simulink model "flatnessLinearNonLinear"  (R2023b)
settings: Solver=FixedStepAuto  StartTime=0.0  StopTime=7  RelTol=1e-3
model workspace (MAT data in the model file):
  kp = Simulink.Parameter
  kp.DataType = 'auto'
  kp.Complexity = 'real'
  kp.Dimensions = [0 0]
libraries: robotmobilelib x2, simulink x1
settings Model: Creator=RichiRettore  LastModifiedBy=RichiRettore

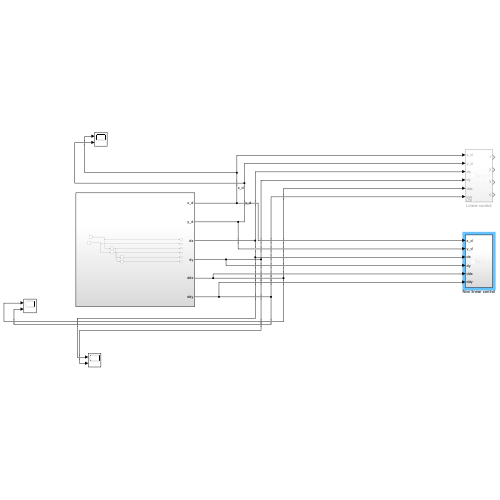
[thumbnail: Simulink's stored preview of the top-level diagram]
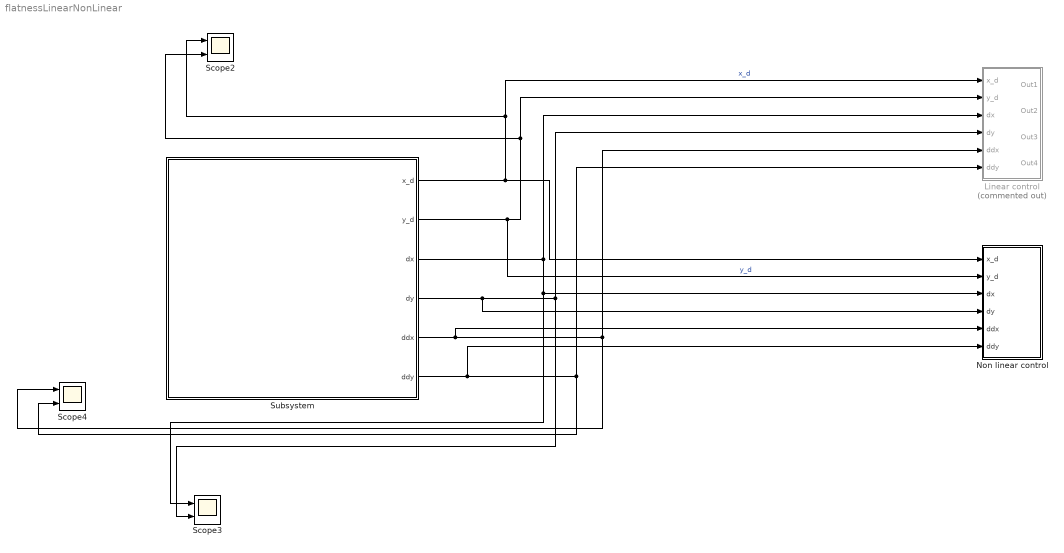
== system flatnessLinearNonLinear ==
  Linear control : Subsystem  Commented=on
  Non linear control : Subsystem
  Scope2 : Scope  NumInputPorts=2
  Scope3 : Scope  NumInputPorts=2
  Scope4 : Scope  NumInputPorts=2
  Subsystem : Subsystem
  wires:
  Subsystem/1(x_d) -> Non linear control/1(x_d), Linear control/1(x_d), Scope2/1  "x_d"
  Subsystem/2(y_d) -> Non linear control/2(y_d), Linear control/2(y_d), Scope2/2  "y_d"
  Subsystem/3(dx) -> Non linear control/3(dx), Scope3/1, Linear control/3(dx)
  Subsystem/4(dy) -> Non linear control/4(dy), Linear control/4(dy), Scope3/2
  Subsystem/5(ddx) -> Non linear control/5(ddx), Linear control/5(ddx), Scope4/1
  Subsystem/6(ddy) -> Non linear control/6(ddy), Linear control/6(ddy), Scope4/2

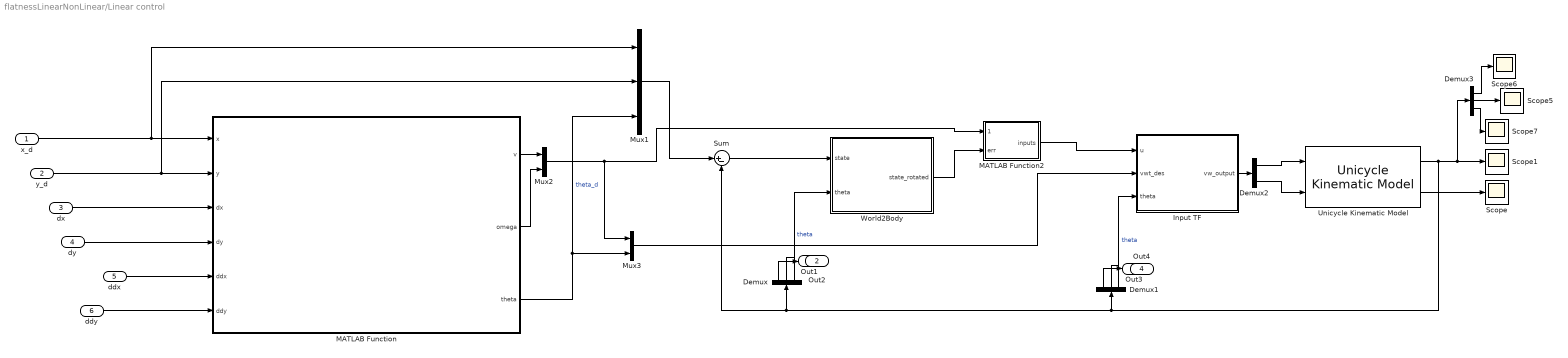
== system flatnessLinearNonLinear/Linear control ==
  x_d : Inport
  y_d : Inport  Port=2
  dx : Inport  Port=3
  dy : Inport  Port=4
  ddx : Inport  Port=5
  ddy : Inport  Port=6
  Demux : Demux  Outputs=3
  Demux1 : Demux  Outputs=3
  Demux2 : Demux  Outputs=2
  Demux3 : Demux  Outputs=3
  Input TF : MATLAB Function  TreatAsAtomicUnit=on
  MATLAB Function : MATLAB Function  TreatAsAtomicUnit=on
  MATLAB Function2 : MATLAB Function  TreatAsAtomicUnit=on
  Mux1 : Mux  Inputs=3
  Mux2 : Mux  Inputs=2
  Mux3 : Mux  Inputs=2
  Scope{,1,5..7} (5 alike) : Scope
  Sum : Sum  Inputs=|+-
  Unicycle Kinematic Model : robotmobilelib/Unicycle Kinematic Model  VehicleInputs=Vehicle Speed & Heading Angular Velocity  WheelRadius=0.1  WheelSpeedRange=[-Inf Inf]  InitialState=[1; 1; 1]  SimulateUsing=Interpreted execution
  World2Body : MATLAB Function  TreatAsAtomicUnit=on
  Out1 : Outport
  Out2 : Outport  Port=2
  Out3 : Outport  Port=3
  Out4 : Outport  Port=4
  wires:
  Demux1/3 -> Input TF/3(theta)  "theta"
  Unicycle Kinematic Model/1 -> Demux3/1, Scope1/1, Sum/2, Demux/1, Demux1/1
  MATLAB Function/2(omega) -> Mux2/2
  dx/1 -> MATLAB Function/3(dx)
  Demux/3 -> World2Body/2(theta)  "theta"
  x_d/1 -> Mux1/1, MATLAB Function/1(x)
  ddx/1 -> MATLAB Function/5(ddx)
  Sum/1 -> World2Body/1(state)
  World2Body/1(state_rotated) -> MATLAB Function2/2(err)
  Demux2/1 -> Unicycle Kinematic Model/1
  MATLAB Function2/1(inputs) -> Input TF/1(u)
  Demux2/2 -> Unicycle Kinematic Model/2
  Demux1/2 -> Out4/1
  Demux/2 -> Out2/1
  Input TF/1(vw_output) -> Demux2/1
  Mux1/1 -> Sum/1
  MATLAB Function/3(theta) -> Mux3/2, Mux1/3  "theta_d"
  y_d/1 -> Mux1/2, MATLAB Function/2(y)
  Demux3/1 -> Scope6/1
  Mux2/1 -> Mux3/1, MATLAB Function2/1(velocities)
  Mux3/1 -> Input TF/2(vwt_des)
  Demux3/3 -> Scope7/1
  Demux3/2 -> Scope5/1
  Unicycle Kinematic Model/2 -> Scope/1
  MATLAB Function/1(v) -> Mux2/1
  ddy/1 -> MATLAB Function/6(ddy)
  dy/1 -> MATLAB Function/4(dy)
  Demux1/1 -> Out3/1
  Demux/1 -> Out1/1

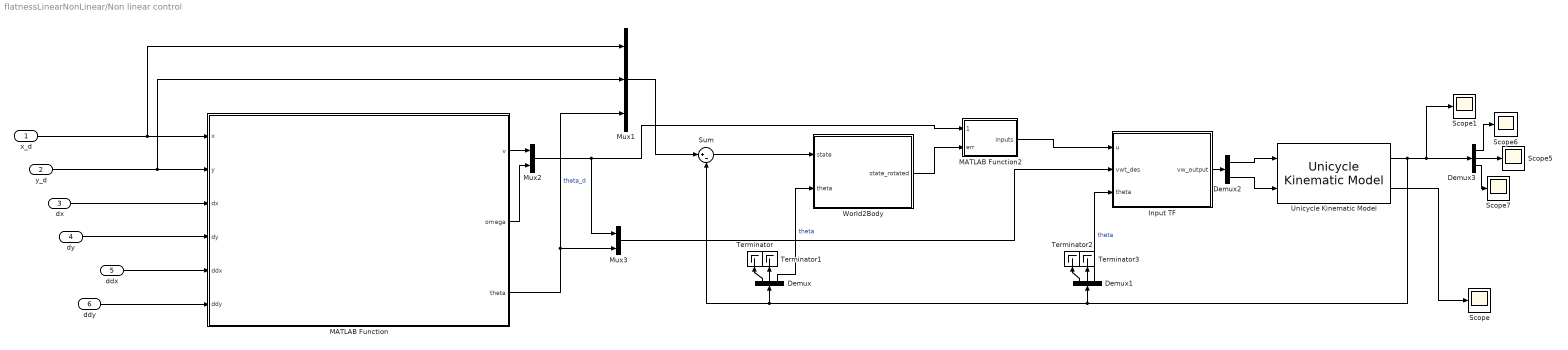
== system flatnessLinearNonLinear/Non linear control ==
  x_d : Inport
  y_d : Inport  Port=2
  dx : Inport  Port=3
  dy : Inport  Port=4
  ddx : Inport  Port=5
  ddy : Inport  Port=6
  Demux : Demux  Outputs=3
  Demux1 : Demux  Outputs=3
  Demux2 : Demux  Outputs=2
  Demux3 : Demux  Outputs=3
  Input TF : MATLAB Function  TreatAsAtomicUnit=on
  MATLAB Function : MATLAB Function  TreatAsAtomicUnit=on
  MATLAB Function2 : MATLAB Function  TreatAsAtomicUnit=on
  Mux1 : Mux  Inputs=3
  Mux2 : Mux  Inputs=2
  Mux3 : Mux  Inputs=2
  Scope{,1,5..7} (5 alike) : Scope
  Sum : Sum  Inputs=|+-
  Terminator{,1..3} (4 alike) : Terminator
  Unicycle Kinematic Model : robotmobilelib/Unicycle Kinematic Model  VehicleInputs=Vehicle Speed & Heading Angular Velocity  WheelRadius=0.1  WheelSpeedRange=[-Inf Inf]  InitialState=[1; 1; 1]  SimulateUsing=Interpreted execution
  World2Body : MATLAB Function  TreatAsAtomicUnit=on
  wires:
  Demux1/3 -> Input TF/3(theta)  "theta"
  Unicycle Kinematic Model/1 -> Demux3/1, Scope1/1, Sum/2, Demux/1, Demux1/1
  MATLAB Function/2(omega) -> Mux2/2
  dx/1 -> MATLAB Function/3(dx)
  Demux/3 -> World2Body/2(theta)  "theta"
  x_d/1 -> Mux1/1, MATLAB Function/1(x)
  ddx/1 -> MATLAB Function/5(ddx)
  Sum/1 -> World2Body/1(state)
  World2Body/1(state_rotated) -> MATLAB Function2/2(err)
  Demux2/1 -> Unicycle Kinematic Model/1
  MATLAB Function2/1(inputs) -> Input TF/1(u)
  Demux2/2 -> Unicycle Kinematic Model/2
  Input TF/1(vw_output) -> Demux2/1
  Mux1/1 -> Sum/1
  MATLAB Function/3(theta) -> Mux3/2, Mux1/3  "theta_d"
  y_d/1 -> Mux1/2, MATLAB Function/2(y)
  Demux3/1 -> Scope6/1
  Mux2/1 -> Mux3/1, MATLAB Function2/1(velocities)
  Mux3/1 -> Input TF/2(vwt_des)
  Demux3/3 -> Scope7/1
  Demux3/2 -> Scope5/1
  Unicycle Kinematic Model/2 -> Scope/1
  MATLAB Function/1(v) -> Mux2/1
  ddy/1 -> MATLAB Function/6(ddy)
  dy/1 -> MATLAB Function/4(dy)
  Demux/2 -> Terminator1/1
  Demux/1 -> Terminator/1
  Demux1/1 -> Terminator2/1
  Demux1/2 -> Terminator3/1

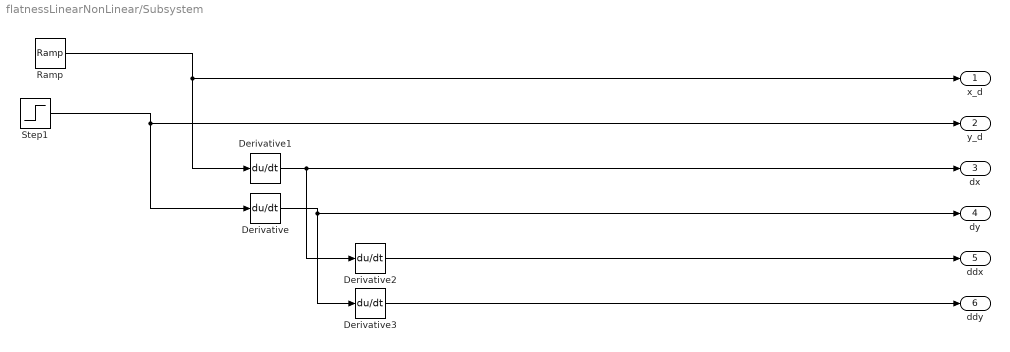
== system flatnessLinearNonLinear/Subsystem ==
  Derivative{,1..3} (4 alike) : Derivative
  Ramp : simulink/Sources/Ramp  slope=1  start=0  InitialOutput=0
  Step1 : Step  Time=0  After=5  SampleTime=0
  x_d : Outport
  y_d : Outport  Port=2
  dx : Outport  Port=3
  dy : Outport  Port=4
  ddx : Outport  Port=5
  ddy : Outport  Port=6
  wires:
  Derivative2/1 -> ddx/1
  Derivative1/1 -> Derivative2/1, dx/1
  Derivative/1 -> Derivative3/1, dy/1
  Step1/1 -> Derivative/1, y_d/1
  Ramp/1 -> Derivative1/1, x_d/1
  Derivative3/1 -> ddy/1

== matlab function flatnessLinearNonLinear/Linear control/World2Body ==
  data: state input; state_rotated output; theta input
function state_rotated = rotation_matrix(state, theta)
% ROTATION_MATRIX Rotates the position [x; y] by an input angle theta.
%
% Inputs:
%   state - 3x1 vector representing [x; y; theta_state]
%   theta - Rotation angle in radians (scalar)
%
% Outputs:
%   state_rotated - 3x1 vector representing the rotated state [x_rot; y_rot; theta_state]

    % Extract x, y, and theta_state from the input state
    x = state(1);
    y = state(2);
    theta_state = state(3);

    % 2D rotation matrix for the x and y components
    R = [cos(theta), sin(theta);
         -sin(theta),  cos(theta)];

    % Rotate the [x; y] part of the state
    xy_rotated = R * [x; y];

    % Combine the rotated x, y, and the original theta_state into a 3x1 vector
    state_rotated = [xy_rotated; theta_state];
end

== matlab function flatnessLinearNonLinear/Linear control/MATLAB Function ==
  data: x input; v output; omega output; y input; theta output; dx input; dy input; ddx input; ddy input
function [v, omega, theta] = unicycle_flatness_num(x, y, dx, dy, ddx, ddy)
    % Compute linear velocity safely
    velocity_magnitude = sqrt(dx^2 + dy^2);
    if velocity_magnitude < 1e-6
        v = 0;
    else
        v = velocity_magnitude;
    end

    % Compute heading angle
    theta = atan2(dy, dx);

    % Compute angular velocity safely
    denominator = dx^2 + dy^2;
    if denominator < 1e-6
        omega = 0;
    else
        omega = (dx * ddy - dy * ddx) / denominator;
    end
end

== matlab function flatnessLinearNonLinear/Linear control/Input TF ==
  data: u input; vwt_des input; vw_output output; theta input
function vw_output = input_transformation(u, vwt_des, theta)
% INPUT_TRANSFORMATION Computes the transformed velocities v and w.
%
% Inputs:
%   u        - 2x1 vector [u1; u2]
%   vwt_des  - 3x1 vector [v_des; w_des; theta_des]
%   theta    - Scalar rotation angle in radians
%
% Outputs:
%   vw_output - 2x1 vector [v; w] representing the transformed velocities

    % Extract inputs
    u1 = u(1);
    u2 = u(2);

    v_des = vwt_des(1);
    w_des = vwt_des(2);
    theta_des = vwt_des(3);

    % Compute the transformed velocities
    v = v_des * cos(theta_des - theta) - u1;
    w = w_des - u2;

    % Combine into a 2x1 output vector
    vw_output = [v; w];
end

== matlab function flatnessLinearNonLinear/Linear control/MATLAB Function2 ==
  data: velocities input; inputs output; err input
function inputs = fcn(velocities, err)
    d = 1 / sqrt(2);
    a = 1;
    vd = velocities(1);
    wd = velocities(2);
    
    % Safeguard for small vd
    vd_safe = sign(vd) * max(abs(vd), 1e-4);
    
    % Gains
    k1 = 2 * d * a;
    k2 = (a^2 - wd^2) / vd_safe;
    k3 = k1;
    
    % Clamp k2 to avoid large values
    max_k2 = 10;
    k2 = max(min(k2, max_k2), -max_k2);
    
    % Gain matrix
    k = [-k1, 0, 0;
         0, -k2, -k3];
    
    % Compute inputs and clamp to avoid excessively large values
    inputs = k * err;
    inputs = max(min(inputs, 10), -10);  % Clamping range for inputs
end

== matlab function flatnessLinearNonLinear/Non linear control/Input TF ==
  data: u input; vwt_des input; vw_output output; theta input
function vw_output = input_transformation(u, vwt_des, theta)
% INPUT_TRANSFORMATION Computes the transformed velocities v and w.
%
% Inputs:
%   u        - 2x1 vector [u1; u2]
%   vwt_des  - 3x1 vector [v_des; w_des; theta_des]
%   theta    - Scalar rotation angle in radians
%
% Outputs:
%   vw_output - 2x1 vector [v; w] representing the transformed velocities

    % Extract inputs
    u1 = u(1);
    u2 = u(2);

    v_des = vwt_des(1);
    w_des = vwt_des(2);
    theta_des = vwt_des(3);

    % Compute the transformed velocities
    v = v_des * cos(theta_des - theta) - u1;
    w = w_des - u2;

    % Combine into a 2x1 output vector
    vw_output = [v; w];
end

== matlab function flatnessLinearNonLinear/Non linear control/MATLAB Function ==
  data: x input; v output; omega output; y input; theta output; dx input; dy input; ddx input; ddy input
function [v, omega, theta] = unicycle_flatness_num(x, y, dx, dy, ddx, ddy)
    % Compute linear velocity safely
    velocity_magnitude = sqrt(dx^2 + dy^2);
    if velocity_magnitude < 1e-6
        v = 0;
    else
        v = velocity_magnitude;
    end

    % Compute heading angle
    theta = atan2(dy, dx);

    % Compute angular velocity safely
    denominator = dx^2 + dy^2;
    if denominator < 1e-6
        omega = 0;
    else
        omega = (dx * ddy - dy * ddx) / denominator;
    end
end

== matlab function flatnessLinearNonLinear/Non linear control/MATLAB Function2 ==
  data: velocities input; inputs output; err input
function inputs = fcn(velocities, err)
    d = 1 / sqrt(2);
    b = 1;
    vd = velocities(1);
    wd = velocities(2);
    e3 = err(3);

    % Safeguard for small vd
    e3 = sign(e3) * max(abs(e3), 1e-4);
    
    % Gains
    k1 = 2 * d * sqrt(b*vd+wd^2);
    k2 = b;
    k3 = k1;
    
    % Gain matrix
    k = [-k1, 0, 0;
         0, -k2*vd*(sin(e3)/e3), -k3];
    
    % Compute inputs and clamp to avoid excessively large values
    inputs = k * err;
    inputs = max(min(inputs, 10), -10);  % Clamping range for inputs
end

== matlab function flatnessLinearNonLinear/Non linear control/World2Body ==
  data: state input; state_rotated output; theta input
function state_rotated = rotation_matrix(state, theta)
% ROTATION_MATRIX Rotates the position [x; y] by an input angle theta.
%
% Inputs:
%   state - 3x1 vector representing [x; y; theta_state]
%   theta - Rotation angle in radians (scalar)
%
% Outputs:
%   state_rotated - 3x1 vector representing the rotated state [x_rot; y_rot; theta_state]

    % Extract x, y, and theta_state from the input state
    x = state(1);
    y = state(2);
    theta_state = state(3);

    % 2D rotation matrix for the x and y components
    R = [cos(theta), sin(theta);
         -sin(theta),  cos(theta)];

    % Rotate the [x; y] part of the state
    xy_rotated = R * [x; y];

    % Combine the rotated x, y, and the original theta_state into a 3x1 vector
    state_rotated = [xy_rotated; theta_state];
end
